simulink model "controller_px4"  (R2018a)
settings: Solver=FixedStepAuto  StartTime=0.0  StopTime=inf  RelTol=1e-3  EnableMultiTasking=on
InitFcn:
  | controller_script
values from neighbouring files (symbols this model uses):
  g = 9.81    [controller_script.m]
  I = [0.06 0.003 0.0006;0.003 0.05 0.002;0.002 0.003 0.1]    [controller_script.m]
  Kp = 15*eye(3)    [controller_script.m]
  Kr = 20*eye(3)    [controller_script.m]
  Kv = 10*eye(3)    [controller_script.m]
  Kw = 2*eye(3)    [controller_script.m]
  m = 1.5    [controller_script.m]
  zw = [0;0;1]    [controller_script.m]
undefined symbols (not defined in the file or in its folder): Orientation, Pose, Thrust, Twist, TypeMask, W, X, Y, Z
libraries: robotlib x14
settings Model: Creator=hugoa  LastModifiedBy=ALEX
settings OptimizationCC: LifeSpan=inf
settings DebuggingCC: SFUnexpectedBacktrackingDiag=warning  SFNoUnconditionalDefaultTransitionDiag=warning  SFExecutionAtInitializationDiag=none
settings CodeAppCC: StateflowObjectComments=on
settings GRTTargetCC: TargetLangStandard=C89/C90 (ANSI)  GeneratePreprocessorConditionals=Disable all
settings ConfigComp: CovMetricSettings=dw  CovHtmlReporting=on  CovSaveCumulativeToWorkspaceVar=on  CovSaveSingleToWorkspaceVar=on  CovExternalEMLEnable=off

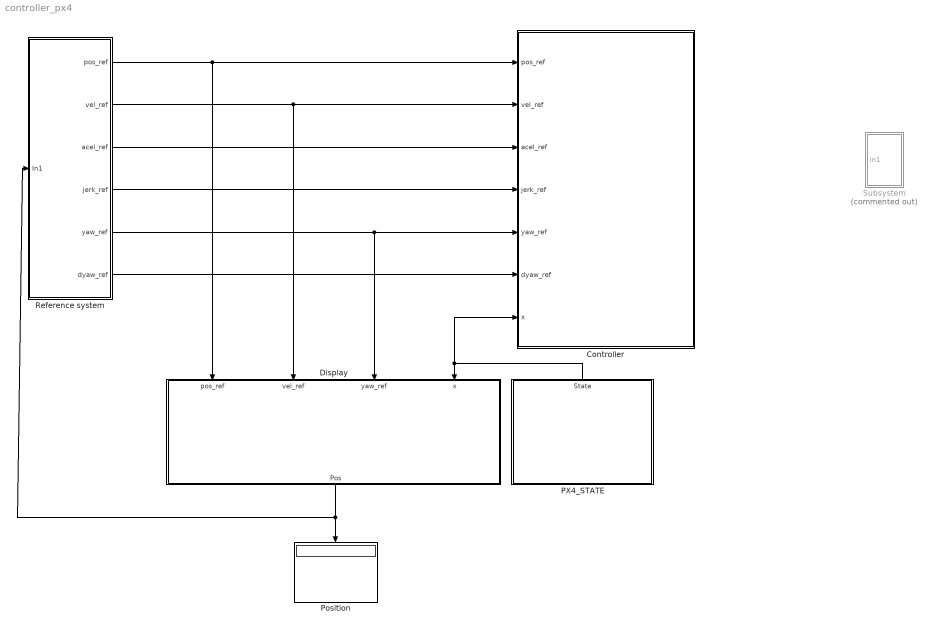
== system controller_px4 ==
  "Controller " : Subsystem
  Display : Subsystem
  "PX4_STATE " : Subsystem
  Position : Display
  Reference system : Subsystem
  Subsystem : Subsystem  Commented=on
  wires:
  Reference system/1(pos_ref) -> Display/1(pos_ref), "Controller "/1(pos_ref)
  Reference system/2(vel_ref) -> Display/2(vel_ref), "Controller "/2(vel_ref)
  Reference system/3(acel_ref) -> "Controller "/3(acel_ref)
  Reference system/4(jerk_ref) -> "Controller "/4(jerk_ref)
  Reference system/5(yaw_ref) -> Display/3(yaw_ref), "Controller "/5(yaw_ref)
  Reference system/6(dyaw_ref) -> "Controller "/6(dyaw_ref)
  "PX4_STATE "/1(State) -> "Controller "/7(x), Display/4(x)
  Display/1(Pos) -> Reference system/1(In1), Position/1

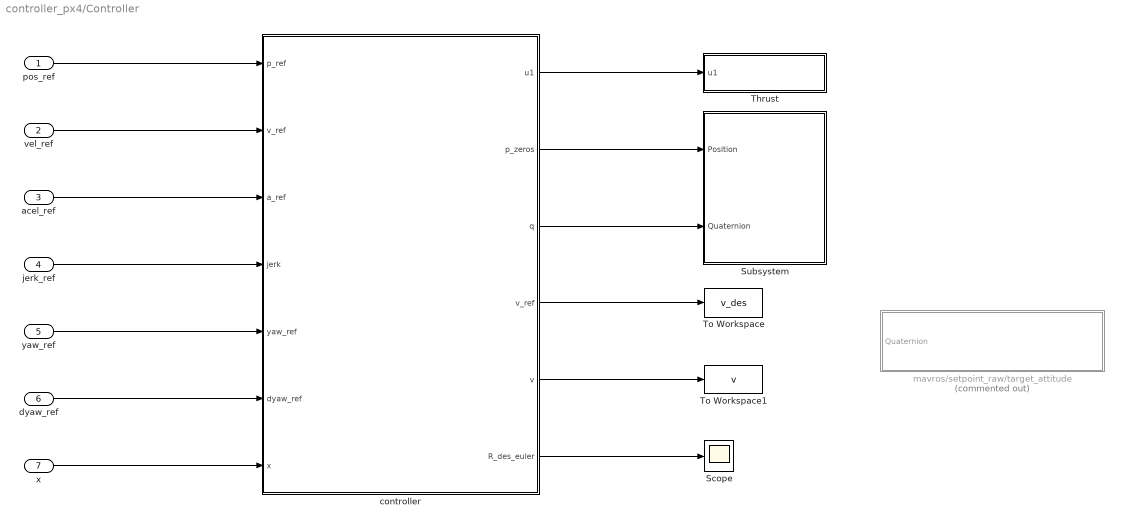
== system controller_px4/Controller  ==
  pos_ref : Inport
  vel_ref : Inport  Port=2
  acel_ref : Inport  Port=3
  jerk_ref : Inport  Port=4
  yaw_ref : Inport  Port=5
  dyaw_ref : Inport  Port=6
  x : Inport  Port=7
  Scope : Scope
  Subsystem : Subsystem
  Thrust : Subsystem
  To Workspace : ToWorkspace  VariableName=v_des  SaveFormat=Timeseries  SampleTime=-1
  To Workspace1 : ToWorkspace  VariableName=v  SaveFormat=Timeseries  SampleTime=-1
  controller : MATLAB Function  TreatAsAtomicUnit=on
  mavros/setpoint_raw/target_attitude : Subsystem  Commented=on
  wires:
  pos_ref/1 -> controller/1(p_ref)
  x/1 -> controller/7(x)
  vel_ref/1 -> controller/2("v_ref ")
  acel_ref/1 -> controller/3(a_ref)
  jerk_ref/1 -> controller/4(jerk)
  yaw_ref/1 -> controller/5(yaw_ref)
  dyaw_ref/1 -> controller/6(dyaw_ref)
  controller/2(p_zeros) -> Subsystem/1(Position)
  controller/1(u1) -> Thrust/1(u1)
  controller/4(v_ref) -> To Workspace/1
  controller/5(v) -> To Workspace1/1
  controller/6(R_des_euler) -> Scope/1
  controller/3(q) -> Subsystem/2(Quaternion)

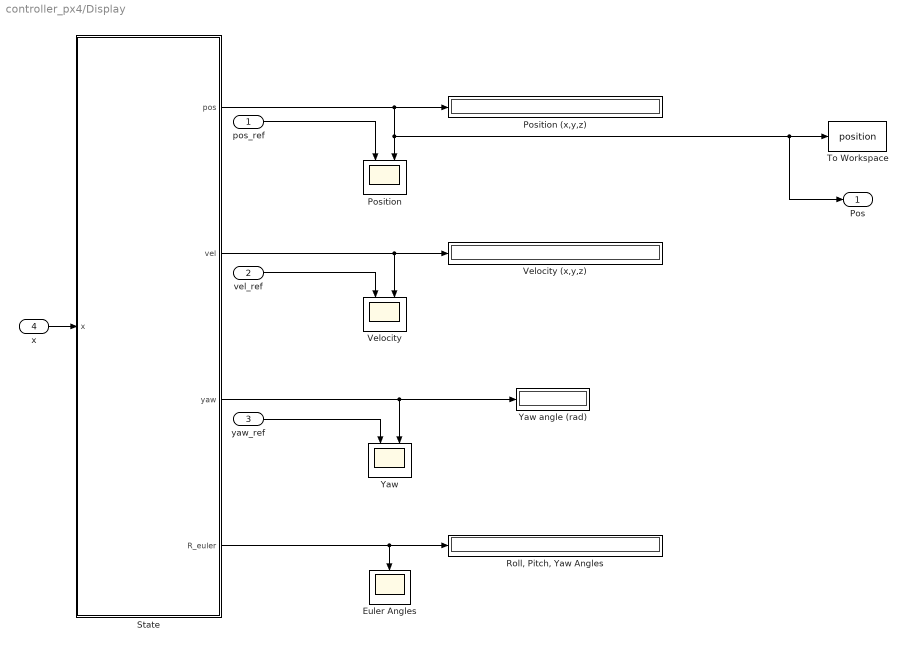
== system controller_px4/Display ==
  pos_ref : Inport
  vel_ref : Inport  Port=2
  yaw_ref : Inport  Port=3
  x : Inport  Port=4
  Euler Angles : Scope
  Position : Scope  NumInputPorts=2
  Position (x,y,z) : Display
  "Roll, Pitch, Yaw Angles" : Display
  State : MATLAB Function  TreatAsAtomicUnit=on
  To Workspace : ToWorkspace  VariableName=position  SaveFormat=Timeseries  SampleTime=-1
  Velocity : Scope  NumInputPorts=2
  Velocity (x,y,z) : Display
  Yaw : Scope  NumInputPorts=2
  Yaw angle (rad) : Display
  Pos : Outport
  wires:
  yaw_ref/1 -> Yaw/1
  x/1 -> State/1(x)
  State/3(yaw) -> Yaw/2, Yaw angle (rad)/1
  State/4(R_euler) -> "Roll, Pitch, Yaw Angles"/1, Euler Angles/1
  vel_ref/1 -> Velocity/1
  State/2(vel) -> Velocity (x,y,z)/1, Velocity/2
  State/1(pos) -> Pos/1, To Workspace/1, Position/2, Position (x,y,z)/1
  pos_ref/1 -> Position/1

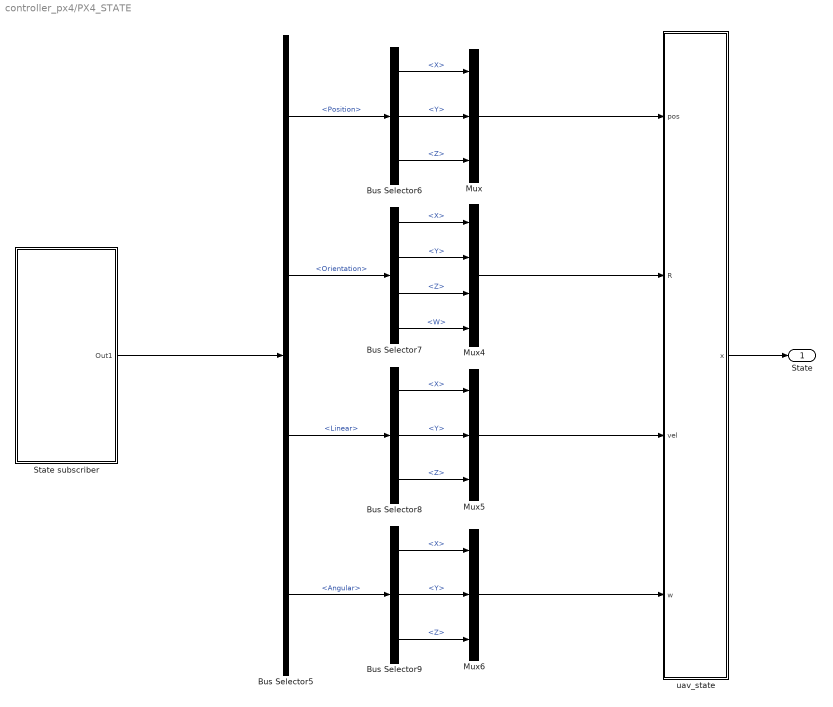
== system controller_px4/PX4_STATE  ==
  Bus Selector5 : BusSelector  OutputSignals=Pose.Pose.Position,Pose.Pose.Orientation,Twist.Twist.Linear,Twist.Twist.Angular
  Bus Selector6 : BusSelector  OutputSignals=X,Y,Z
  Bus Selector7 : BusSelector  OutputSignals=X,Y,Z,W
  Bus Selector8 : BusSelector  OutputSignals=X,Y,Z
  Bus Selector9 : BusSelector  OutputSignals=X,Y,Z
  Mux : Mux  Inputs=3
  Mux4 : Mux
  Mux5 : Mux  Inputs=3
  Mux6 : Mux  Inputs=3
  State subscriber : Subsystem
  uav_state : MATLAB Function  TreatAsAtomicUnit=on
  State : Outport
  wires:
  Bus Selector5/1 -> Bus Selector6/1  "<Position>"
  Bus Selector7/3 -> Mux4/3  "<Z>"
  Bus Selector7/1 -> Mux4/1  "<X>"
  Bus Selector5/3 -> Bus Selector8/1  "<Linear>"
  Bus Selector8/1 -> Mux5/1  "<X>"
  Bus Selector5/4 -> Bus Selector9/1  "<Angular>"
  Bus Selector9/2 -> Mux6/2  "<Y>"
  Bus Selector7/4 -> Mux4/4  "<W>"
  Bus Selector9/1 -> Mux6/1  "<X>"
  Bus Selector7/2 -> Mux4/2  "<Y>"
  Bus Selector8/2 -> Mux5/2  "<Y>"
  Bus Selector8/3 -> Mux5/3  "<Z>"
  Bus Selector9/3 -> Mux6/3  "<Z>"
  Bus Selector5/2 -> Bus Selector7/1  "<Orientation>"
  uav_state/1(x) -> State/1
  Bus Selector6/1 -> Mux/1  "<X>"
  Bus Selector6/2 -> Mux/2  "<Y>"
  Bus Selector6/3 -> Mux/3  "<Z>"
  Mux/1 -> uav_state/1(pos)
  Mux5/1 -> uav_state/3(vel)
  Mux6/1 -> uav_state/4(w)
  Mux4/1 -> uav_state/2(R)
  State subscriber/1(Out1) -> Bus Selector5/1

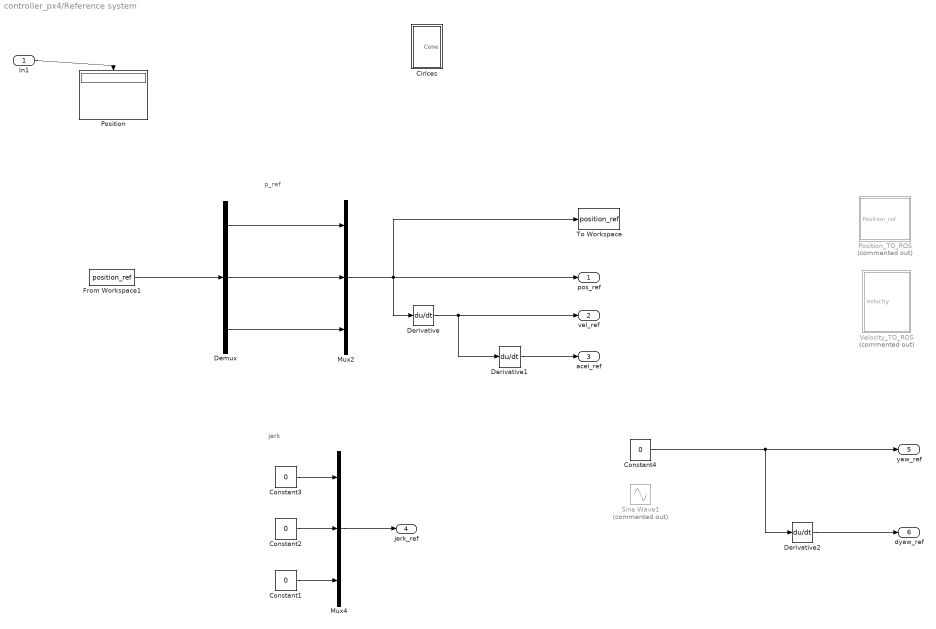
== system controller_px4/Reference system ==
  note: jerk
  note: p_ref
  In1 : Inport
  Cirlces : Subsystem
  Constant{1..4} (4 alike) : Constant  Value=0
  Demux : Demux  Outputs=3
  Derivative : Derivative  CoefficientInTFapproximation=0.01
  Derivative1 : Derivative  CoefficientInTFapproximation=0.01
  Derivative2 : Derivative  CoefficientInTFapproximation=0.01
  From Workspace1 : FromWorkspace  VariableName=position_ref  SampleTime=0
  Mux2 : Mux  Inputs=3
  Mux4 : Mux  Inputs=3
  Position : Display
  Position_TO_ROS : Subsystem  Commented=on
  Sine Wave1 : Sin  Commented=on  SampleTime=0
  To Workspace : ToWorkspace  VariableName=position_ref  SaveFormat=Timeseries  SampleTime=-1
  Velocity_TO_ROS : Subsystem  Commented=on
  pos_ref : Outport
  vel_ref : Outport  Port=2
  acel_ref : Outport  Port=3
  jerk_ref : Outport  Port=4
  yaw_ref : Outport  Port=5
  dyaw_ref : Outport  Port=6
  wires:
  Constant4/1 -> Derivative2/1, yaw_ref/1
  Constant3/1 -> Mux4/1
  Constant1/1 -> Mux4/3
  Constant2/1 -> Mux4/2
  Derivative/1 -> vel_ref/1, Derivative1/1
  Derivative1/1 -> acel_ref/1
  Derivative2/1 -> dyaw_ref/1
  Mux4/1 -> jerk_ref/1
  In1/1 -> Position/1
  Demux/3 -> Mux2/3
  Demux/2 -> Mux2/2
  Demux/1 -> Mux2/1
  From Workspace1/1 -> Demux/1
  Mux2/1 -> pos_ref/1, To Workspace/1, Derivative/1

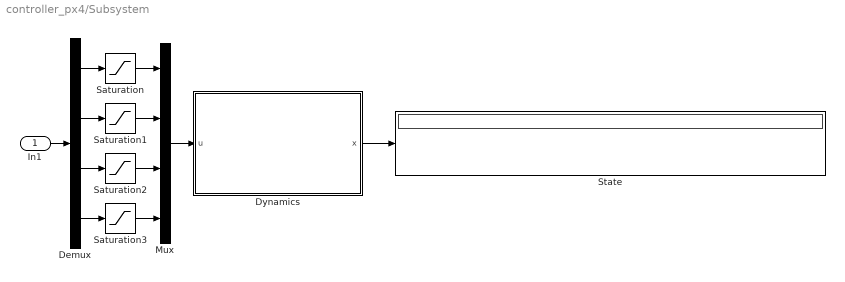
== system controller_px4/Subsystem ==
  In1 : Inport
  Demux : Demux
  Dynamics : Subsystem
  Mux : Mux
  Saturation : Saturate  UpperLimit=1000  LowerLimit=-100
  Saturation1 : Saturate  UpperLimit=1000  LowerLimit=-100
  Saturation2 : Saturate  UpperLimit=100  LowerLimit=-100
  Saturation3 : Saturate  UpperLimit=100  LowerLimit=-100
  State : Display
  wires:
  Demux/3 -> Saturation2/1
  Mux/1 -> Dynamics/1(u)
  Dynamics/1(x) -> State/1
  In1/1 -> Demux/1
  Demux/4 -> Saturation3/1
  Saturation3/1 -> Mux/4
  Saturation1/1 -> Mux/2
  Demux/1 -> Saturation/1
  Saturation/1 -> Mux/1
  Demux/2 -> Saturation1/1
  Saturation2/1 -> Mux/3

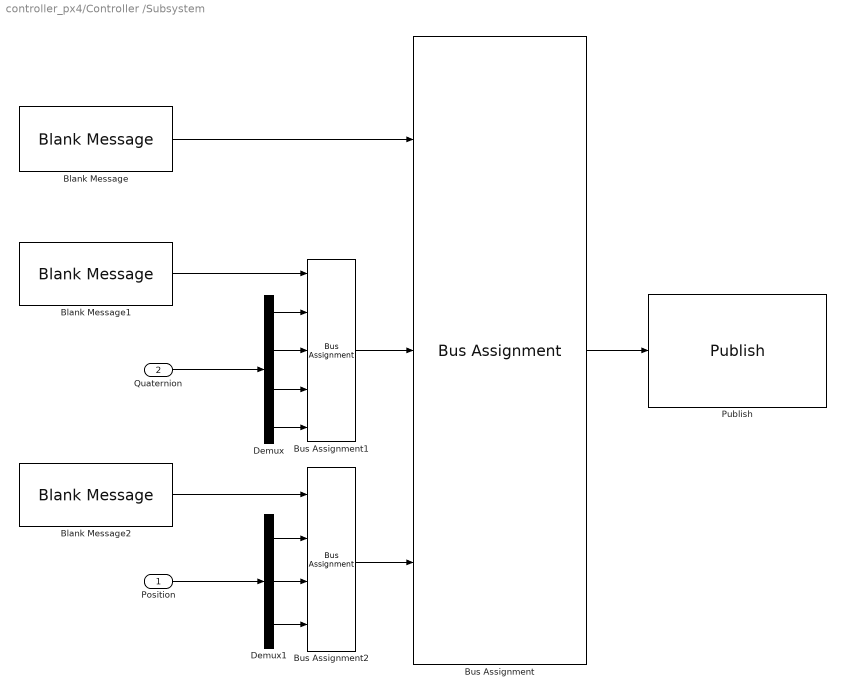
== system controller_px4/Controller /Subsystem ==
  Position : Inport
  Quaternion : Inport  Port=2
  Blank Message : robotlib/Blank Message  SourceLibraryInfo=This block requires Robotics System Toolbox  messageType=geometry_msgs/PoseStamped  SampleTime=inf
      settings: SourceProductBaseCode=RO
  Blank Message1 : robotlib/Blank Message  SourceLibraryInfo=This block requires Robotics System Toolbox  messageType=geometry_msgs/Quaternion  SampleTime=inf
      settings: SourceProductBaseCode=RO
  Blank Message2 : robotlib/Blank Message  SourceLibraryInfo=This block requires Robotics System Toolbox  messageType=geometry_msgs/Point  SampleTime=inf
      settings: SourceProductBaseCode=RO
  Bus Assignment : BusAssignment  AssignedSignals=Pose.Orientation,Pose.Position
  Bus Assignment1 : BusAssignment  AssignedSignals=W,X,Y,Z
  Bus Assignment2 : BusAssignment  AssignedSignals=X,Y,Z
  Demux : Demux
  Demux1 : Demux  Outputs=3
  Publish : robotlib/Publish  SourceLibraryInfo=This block requires Robotics System Toolbox  topicSource=Specify your own  topic=/sim_attitude  messageType=geometry_msgs/PoseStamped  messageQueueLength=1
      settings: SourceProductBaseCode=RO
  wires:
  Bus Assignment1/1 -> Bus Assignment/2
  Blank Message1/1 -> Bus Assignment1/1
  Bus Assignment/1 -> Publish/1
  Blank Message/1 -> Bus Assignment/1
  Quaternion/1 -> Demux/1
  Blank Message2/1 -> Bus Assignment2/1
  Demux1/1 -> Bus Assignment2/2
  Demux1/3 -> Bus Assignment2/4
  Demux1/2 -> Bus Assignment2/3
  Position/1 -> Demux1/1
  Bus Assignment2/1 -> Bus Assignment/3
  Demux/1 -> Bus Assignment1/2
  Demux/2 -> Bus Assignment1/3
  Demux/3 -> Bus Assignment1/4
  Demux/4 -> Bus Assignment1/5

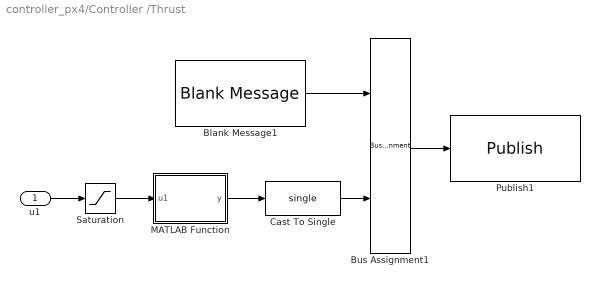
== system controller_px4/Controller /Thrust ==
  u1 : Inport
  Blank Message1 : robotlib/Blank Message  SourceLibraryInfo=This block requires Robotics System Toolbox  messageType=std_msgs/Float32  SampleTime=inf
      settings: SourceProductBaseCode=RO
  Bus Assignment1 : BusAssignment  AssignedSignals=Data
  Cast To Single : DataTypeConversion  OutDataTypeStr=single
  MATLAB Function : MATLAB Function  TreatAsAtomicUnit=on
  Publish1 : robotlib/Publish  SourceLibraryInfo=This block requires Robotics System Toolbox  topicSource=Specify your own  topic=/sim_thrust  messageType=std_msgs/Float32  messageQueueLength=1
      settings: SourceProductBaseCode=RO
  Saturation : Saturate  UpperLimit=20  LowerLimit=0
  wires:
  Blank Message1/1 -> Bus Assignment1/1
  Bus Assignment1/1 -> Publish1/1
  Cast To Single/1 -> Bus Assignment1/2
  MATLAB Function/1(y) -> Cast To Single/1
  u1/1 -> Saturation/1
  Saturation/1 -> MATLAB Function/1(u1)

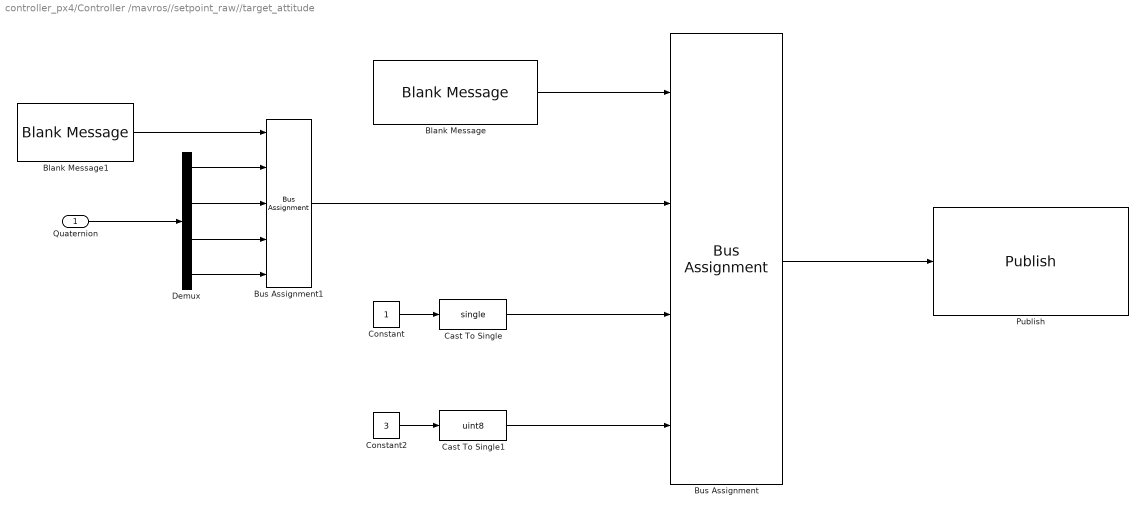
== system controller_px4/Controller /mavros//setpoint_raw//target_attitude ==
  Quaternion : Inport
  Blank Message : robotlib/Blank Message  SourceLibraryInfo=This block requires Robotics System Toolbox  messageType=mavros_msgs/AttitudeTarget  SampleTime=inf
      settings: SourceProductBaseCode=RO
  Blank Message1 : robotlib/Blank Message  SourceLibraryInfo=This block requires Robotics System Toolbox  messageType=geometry_msgs/Quaternion  SampleTime=inf
      settings: SourceProductBaseCode=RO
  Bus Assignment : BusAssignment  AssignedSignals=Orientation,Thrust,TypeMask
  Bus Assignment1 : BusAssignment  AssignedSignals=X,Y,Z,W
  Cast To Single : DataTypeConversion  OutDataTypeStr=single
  Cast To Single1 : DataTypeConversion  OutDataTypeStr=uint8
  Constant : Constant
  Constant2 : Constant  Value=3
  Demux : Demux
  Publish : robotlib/Publish  SourceLibraryInfo=This block requires Robotics System Toolbox  topicSource=Specify your own  topic=/mavros/setpoint_raw/target_attitude  messageType=mavros_msgs/AttitudeTarget  messageQueueLength=1
      settings: SourceProductBaseCode=RO
  wires:
  Bus Assignment1/1 -> Bus Assignment/2
  Demux/3 -> Bus Assignment1/4
  Blank Message1/1 -> Bus Assignment1/1
  Demux/4 -> Bus Assignment1/5
  Bus Assignment/1 -> Publish/1
  Demux/1 -> Bus Assignment1/2
  Cast To Single/1 -> Bus Assignment/3
  Blank Message/1 -> Bus Assignment/1
  Constant/1 -> Cast To Single/1
  Demux/2 -> Bus Assignment1/3
  Quaternion/1 -> Demux/1
  Cast To Single1/1 -> Bus Assignment/4
  Constant2/1 -> Cast To Single1/1

== system controller_px4/PX4_STATE /State subscriber ==
  Subscribe : robotlib/Subscribe  SourceLibraryInfo=This block requires Robotics System Toolbox  topicSource=Specify your own  topic=/mavros/local_position/odom  messageType=nav_msgs/Odometry  sampleTime=-1  messageQueueLength=1
      settings: SourceProductBaseCode=RO
  Terminator : Terminator
  Out1 : Outport
  wires:
  Subscribe/1 -> Terminator/1
  Subscribe/2 -> Out1/1

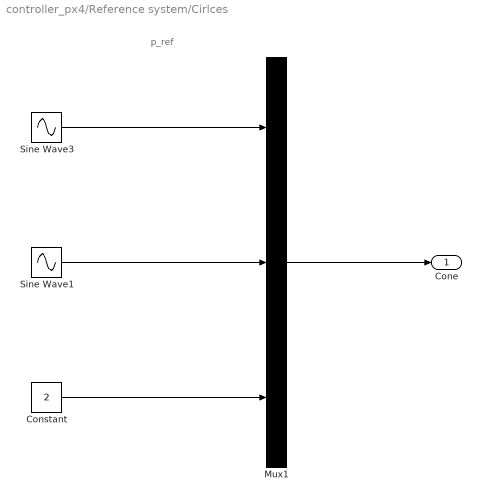
== system controller_px4/Reference system/Cirlces ==
  note: p_ref
  Constant : Constant  Value=2
  Mux1 : Mux  Inputs=3
  Sine Wave1 : Sin  Amplitude=2  Frequency=2  Phase=pi/2  SampleTime=0
  Sine Wave3 : Sin  Amplitude=2  Frequency=2  SampleTime=0
  Cone : Outport
  wires:
  Sine Wave1/1 -> Mux1/2
  Constant/1 -> Mux1/3
  Sine Wave3/1 -> Mux1/1
  Mux1/1 -> Cone/1

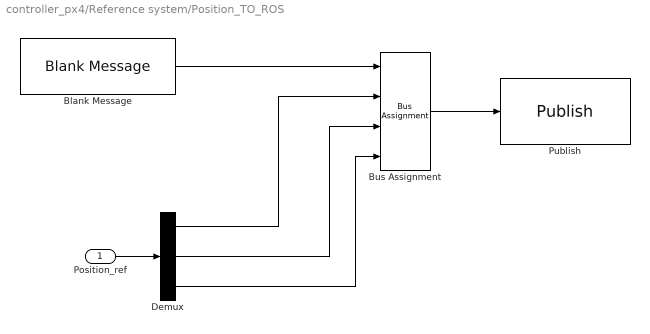
== system controller_px4/Reference system/Position_TO_ROS ==
  Position_ref : Inport
  Blank Message : robotlib/Blank Message  SourceLibraryInfo=This block requires Robotics System Toolbox  messageType=geometry_msgs/PoseStamped  SampleTime=inf
      settings: SourceProductBaseCode=RO
  Bus Assignment : BusAssignment  AssignedSignals=Pose.Position.X,Pose.Position.Y,Pose.Position.Z
  Demux : Demux  Outputs=3
  Publish : robotlib/Publish  SourceLibraryInfo=This block requires Robotics System Toolbox  topicSource=Specify your own  topic=/sim_position  messageType=geometry_msgs/PoseStamped  messageQueueLength=1
      settings: SourceProductBaseCode=RO
  wires:
  Blank Message/1 -> Bus Assignment/1
  Bus Assignment/1 -> Publish/1
  Demux/1 -> Bus Assignment/2
  Demux/2 -> Bus Assignment/3
  Demux/3 -> Bus Assignment/4
  Position_ref/1 -> Demux/1

== system controller_px4/Reference system/Velocity_TO_ROS ==
  Velocity : Inport
  Blank Message1 : robotlib/Blank Message  SourceLibraryInfo=This block requires Robotics System Toolbox  messageType=geometry_msgs/TwistStamped  SampleTime=inf
      settings: SourceProductBaseCode=RO
  Bus Assignment1 : BusAssignment  AssignedSignals=Twist.Linear.X,Twist.Linear.Y,Twist.Linear.Z
  Demux2 : Demux  Outputs=3
  Publish1 : robotlib/Publish  SourceLibraryInfo=This block requires Robotics System Toolbox  topicSource=Specify your own  topic=/my_vel  messageType=geometry_msgs/TwistStamped  messageQueueLength=1
      settings: SourceProductBaseCode=RO
  wires:
  Bus Assignment1/1 -> Publish1/1
  Demux2/2 -> Bus Assignment1/3
  Demux2/1 -> Bus Assignment1/2
  Blank Message1/1 -> Bus Assignment1/1
  Demux2/3 -> Bus Assignment1/4
  Velocity/1 -> Demux2/1

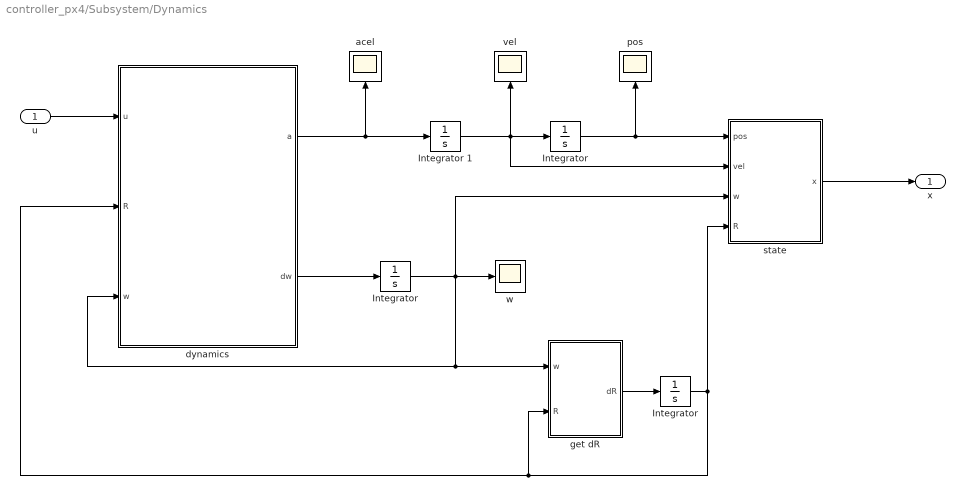
== system controller_px4/Subsystem/Dynamics ==
  u : Inport
  "Integrator " : Integrator  InitialCondition=eye(3)  UpperSaturationLimit=1  LowerSaturationLimit=0
  "Integrator " : Integrator  InitialCondition=[0;0;0]
  "Integrator " : Integrator  InitialCondition=[0;0;0]
  Integrator 1 : Integrator  InitialCondition=[0;0;0]
  acel : Scope
  dynamics : MATLAB Function  TreatAsAtomicUnit=on
  get dR : MATLAB Function  TreatAsAtomicUnit=on
  pos : Scope
  state : MATLAB Function  TreatAsAtomicUnit=on
  vel : Scope
  w : Scope
  x : Outport
  wires:
  dynamics/2(dw) -> "Integrator "/1
  dynamics/1(a) -> Integrator 1/1, acel/1
  "Integrator "/1 -> state/3(w), w/1, dynamics/3(w), get dR/1(w)
  Integrator 1/1 -> vel/1, "Integrator "/1, state/2(vel)
  "Integrator "/1 -> pos/1, state/1(pos)
  "Integrator "/1 -> dynamics/2(R), get dR/2(R), state/4(R)
  state/1(x) -> x/1
  get dR/1(dR) -> "Integrator "/1
  u/1 -> dynamics/1(u)

== matlab function controller_px4/Subsystem/Dynamics/get dR ==
  data: dR output; w input; R input
function dR = fcn(w, R)
%#codegen
skew_w = [0,-w(3),w(2); w(3),0,-w(1); -w(2),w(1),0];



dR = R*skew_w;

== matlab function controller_px4/Subsystem/Dynamics/dynamics ==
  data: u input; R input; a output; w input size=3; dw output; I parameter; g parameter; m parameter
function [a,dw] = fcn(u,R,w, I, g, m)
%#codegen
zw = [0;0;1];
zB = R*zw;

skew_w = [0,-w(3),w(2); w(3),0,-w(1); -w(2),w(1),0];
uT = [u(2);u(3);u(4)];



a = -g*zw+(u(1)/m)*zB;
%dw = inv(I)*(-skew_w*I*w + uT);
dw = I\((cross(-w,I*w))+uT);

== matlab function controller_px4/Subsystem/Dynamics/state ==
  data: pos input; vel input; w input; R input; x output
function x = fcn(pos, vel, w, R)
%#codegen

x = [pos, vel, w, R];

== matlab function controller_px4/Controller /controller ==
  data: p_ref input; v_ref input; a_ref input; jerk input; yaw_ref input; dyaw_ref input; u1 output; x input; Kp parameter; g parameter; Kr parameter; m parameter; zw parameter; Kv parameter; Kw parameter; p_zeros output; q output; v_ref output; v output; R_des_euler output
function [u1, p_zeros, q, v_ref, v, R_des_euler]    = fcn(p_ref, v_ref, a_ref, jerk, yaw_ref, dyaw_ref, x, Kp, g, Kr, m, zw, Kv, Kw)

%% GET THE STATE
    %Position
    p = x(1:3,1);
    %Velocity
    v = x(1:3,2);
    %Angular velocity
    wb = x(1:3,3);
    %Rotation matrix
    R = x(1:3,4:6);
    %R_euler = rotm2eul(R);
    p_zeros = [0;0;0];
    
    % Ganhos estáticos para melhorar os resultados
    ganho_estatico_Z = 3.45;
    ganho_estatico_XY = 0.15;
    
    p_ref(1) = p_ref(1) + ganho_estatico_XY;
    p_ref(2) = p_ref(2) + ganho_estatico_XY;
    p_ref(3) = p_ref(3) - ganho_estatico_Z;
%%%%%%%%%%%%%%%%%%%%%%%%%%%%%%%%%%%%%%%%%%%%%%%

%% ERRORS

    %Position Error
    ep = p - p_ref;
    %Velocity Error
    ev = v - v_ref;

%%%%%%%%%%%%%%%%%%%%%%%%%%%%%%%%%%%%%%%%%%%%%%%

%% EQUATIONS

    F_des   = -Kp*ep - Kv*ev + m*g*zw + m*a_ref;

    zB      = R*zw;
    u1      = dot(F_des, zB);

    %Rotation matrix
    zB_des  = F_des/norm(F_des);
    xA_des  = [cos(yaw_ref); sin(yaw_ref); 0];
    yB_des  = cross(zB_des,xA_des)/norm(cross(zB_des,xA_des));
    xB_des  = cross(yB_des,zB_des);
    R_des   = [xB_des, yB_des, zB_des];
    
    %Orientation Error
    eR_aux  = (transpose(R_des)*R - transpose(R)*R_des);
    eR      = 0.5 * [eR_aux(3,2); eR_aux(1,3); eR_aux(2,1)];

    %Angular velocity
    h       = m/u1*(jerk - ( dot(zB_des, jerk)*zB_des));
    p_des   = dot(-h,yB_des);
    q_des   = dot(h,xB_des);
    % VERY BAD
    w_aux   = R\[xA_des yB_des zw]*[0;0;dyaw_ref];
    r_des   = w_aux(3);

    wb_ref  = [p_des; q_des; r_des];
    
    %Angular Velocity Error
    ew      = wb - wb_ref; 

    
%%%%%%%%%%%%%%%%%%%%%%%%%%%%%%%%%%%%%%%%%%%%%%%

%% Limit yaw angle to pi/6 = 30º
    R_des_euler = rotm2eul(R_des);
    if(R_des_euler(3)>pi/6)
        R_des_euler(3) = pi/6;
    end
    if(R_des_euler(3)<-pi/6)
        R_des_euler(3) = -pi/6;
    end

%% OUTPUT

    uT = - Kr*eR - Kw*ew;
    u = [u1; uT];
    q = eul2quat(R_des_euler);   
%%%%%%%%%%%%%%%%%%%%%%%%%%%%%%%%%%%%%%%%%%%%%%%

== matlab function controller_px4/Display/State ==
  data: x input; pos output; vel output; yaw output; R_euler output
function [pos, vel, yaw, R_euler] = fcn(x)
%#codegen


 R = x(1:3,4:6);
 R_euler_aux = rotm2eul(R);
 %R_euler(1)    ->  Z   ->  Yaw
 %R_euler(2)    ->  X   ->  Roll
 %R_euler(3)    ->  Y   ->  Pitch
 R_euler = [R_euler_aux(2); R_euler_aux(3); R_euler_aux(1)];
 
 
% OUTPUT
pos = x(1:3,1);
vel = x(1:3,2);
yaw = R_euler(3);

== matlab function controller_px4/PX4_STATE /uav_state ==
  data: pos input; R input; vel input; w input; x output
function x = fcn(pos, R, vel, w)
%#codegen
R_euler = quat2rotm(transpose(R));

x = [pos, vel, w, R_euler];

== matlab function controller_px4/Controller /Thrust/MATLAB Function ==
  data: u1 input; y output
function y = fcn(u1)

y = u1/20;
